simulink model "Utkarsh_2005574_R_W3_P2"  (R2021a)
settings: Solver=VariableStepAuto  StartTime=0.0  StopTime=10.0  RelTol=1e-3
settings Model: Creator=Utkarsh Anand  LastModifiedBy=Utkarsh Anand

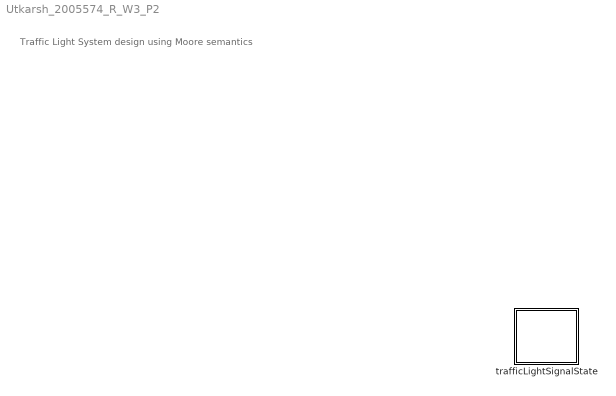
== system Utkarsh_2005574_R_W3_P2 ==
  note: Traffic Light System design using Moore semantics
  trafficLightSignalState : Stateflow chart  TreatAsAtomicUnit=on

== stateflow chart Utkarsh_2005574_R_W3_P2/trafficLightSignalState ==
  state initialStandsill
    northSouth1=red;
    eastWest2=green;
  state haltForTraffic
    northSouth1=red;
    eastWest2=green;
  (default) -> initialStandsill
